simulink model "justina_control"  (R2020a)
settings: Solver=ode4  StartTime=0.0  StopTime=inf  FixedStep=0.004  MaxStep=0.01  RelTol=1e-3
PreLoadFcn:
  | load('justina_rigid_body_tree')
InitFcn:
  | [lowpass_B, lowpass_A] = butter(4,1,'s');
  | manipulator_tree = importrobot('justina_description.urdf');
  | manipulator_tree.Gravity = [9.81 0 0];
model workspace (MAT data in the model file):
  SL_ROS_VariableLengthArrays_MaxSizes.CommonInfo.ArrayTruncateAction = 'EmitWarning'
  SL_ROS_VariableLengthArrays_MaxSizes.MsgTypeMap = containers.Map
  SL_ROS_VariableLengthArrays_MaxSizes.MsgTypeMap.serialization.keys = {'sensor_msgs/JointState', 'std_msgs/Float32MultiArray', 'std_msgs/Float64MultiArray', 'std_msgs/String'}
  SL_ROS_VariableLengthArrays_MaxSizes.MsgTypeMap.serialization.values{1}(1).PropertyName = 'Effort'
  SL_ROS_VariableLengthArrays_MaxSizes.MsgTypeMap.serialization.values{1}(1).DataType = 'double'
  SL_ROS_VariableLengthArrays_MaxSizes.MsgTypeMap.serialization.values{1}(1).MaxLength = 7
  SL_ROS_VariableLengthArrays_MaxSizes.MsgTypeMap.serialization.values{1}(2).PropertyName = 'Name'
  SL_ROS_VariableLengthArrays_MaxSizes.MsgTypeMap.serialization.values{1}(2).DataType = 'std_msgs/String'
  SL_ROS_VariableLengthArrays_MaxSizes.MsgTypeMap.serialization.values{1}(2).MaxLength = 7
  SL_ROS_VariableLengthArrays_MaxSizes.MsgTypeMap.serialization.values{1}(3).PropertyName = 'Position'
  SL_ROS_VariableLengthArrays_MaxSizes.MsgTypeMap.serialization.values{1}(3).DataType = 'double'
  SL_ROS_VariableLengthArrays_MaxSizes.MsgTypeMap.serialization.values{1}(3).MaxLength = 7
  SL_ROS_VariableLengthArrays_MaxSizes.MsgTypeMap.serialization.values{1}(4).PropertyName = 'Velocity'
  SL_ROS_VariableLengthArrays_MaxSizes.MsgTypeMap.serialization.values{1}(4).DataType = 'double'
  SL_ROS_VariableLengthArrays_MaxSizes.MsgTypeMap.serialization.values{1}(4).MaxLength = 7
  SL_ROS_VariableLengthArrays_MaxSizes.MsgTypeMap.serialization.values{2}.PropertyName = 'Data'
  SL_ROS_VariableLengthArrays_MaxSizes.MsgTypeMap.serialization.values{2}.DataType = 'single'
  SL_ROS_VariableLengthArrays_MaxSizes.MsgTypeMap.serialization.values{2}.MaxLength = 14
  SL_ROS_VariableLengthArrays_MaxSizes.MsgTypeMap.serialization.values{3}.PropertyName = 'Data'
  SL_ROS_VariableLengthArrays_MaxSizes.MsgTypeMap.serialization.values{3}.DataType = 'double'
  SL_ROS_VariableLengthArrays_MaxSizes.MsgTypeMap.serialization.values{3}.MaxLength = 7
  SL_ROS_VariableLengthArrays_MaxSizes.MsgTypeMap.serialization.values{4}.PropertyName = 'Data'
  SL_ROS_VariableLengthArrays_MaxSizes.MsgTypeMap.serialization.values{4}.DataType = 'uint8'
  SL_ROS_VariableLengthArrays_MaxSizes.MsgTypeMap.serialization.values{4}.MaxLength = 10
  SL_ROS_VariableLengthArrays_MaxSizes.MsgTypeMap.serialization.uniformity = 0
  SL_ROS_VariableLengthArrays_MaxSizes.MsgTypeMap.serialization.keyType = 'char'
  SL_ROS_VariableLengthArrays_MaxSizes.MsgTypeMap.serialization.valueType = 'any'
undefined symbols (not defined in the file or in its folder): Data, Data_SL_Info
libraries: robotlib x19, robotmaniplib x1
settings Model: EnablePacing=on  Creator=marco  LastModifiedBy=josea
settings OptimizationCC: EnhancedBackFolding=on  PassReuseOutputArgsAs=Individual arguments  ZeroExternalMemoryAtStartup=off  ZeroInternalMemoryAtStartup=off  MaxStackSize=64  OptimizeBlockOrder=speed  DifferentSizesBufferReuse=on  OptimizationCustomize=off  EfficientTunableParamExpr=on
settings DebuggingCC: ParameterTunabilityLossMsg=error
settings HardwareCC: ProdBitPerLong=64  ProdHWDeviceType=Intel->x86-64 (Linux 64)
settings SFSimCC: CustomCodeUndefinedFunction=ThrowError
settings RTWCC: SystemTargetFile=ert.tlc  HardwareBoard=Robot Operating System (ROS)  TemplateMakefile=ert_default_tmf  GenerateReport=on  Toolchain=Catkin  IncludeHyperlinkInReport=on  LaunchReport=on  TargetLang=C++  GenerateTraceInfo=on  GenerateTraceReport=on  GenerateTraceReportSl=on  GenerateTraceReportSf=on  GenerateTraceReportEml=on
settings CodeAppCC: ForceParamTrailComments=on  IgnoreCustomStorageClasses=off  OperatorAnnotations=on  SimulinkDataObjDesc=on  SFDataObjDesc=on  InsertBlockDesc=on
settings ERTTargetCC: SupportContinuousTime=on  SupportVariableSizeSignals=on
settings ExplorerConfigSet: InternalSimMechanicsExplorerSettings="<ExplorerConfiguration><canonicalview>aerospace</canonicalview><AnimationSetting><BasePlaybackSpeed>1.0</BasePlaybackSpeed><PlaybackSpeedFactor>1.0</PlaybackSpeedFactor></AnimationSetting><TilePanel><TileInfo><Tiles Columns=\"1\" Count=\"1\" Rows=\"1\"><Column Weight=\"1\"/><Row Weight=\"1\"/><Tile Height=\"1\" Width=\"1\" X=\"0\" Y=\"0\"/></Tiles></TileInfo><SceneInfo><SceneViewer><BGColor><R>0.60000002384185791</R><G>0.60000002384185791</G><B>0.60000002384185791</B></BGColor><Camera><DoPerspective>off</DoPerspective><Position><X>0.470747241724220999</X><Y>0.672742710715300452</Y><Z>0.803552756362765797</Z></Position><Center><X>0.426167977285198674</X><Y>0.0857009724355916047</Y><Z>-0.00477557216445684274</Z></Center><Up><X>-0.998971998504803671</X><Y>0.0328560329609175472</Y><Z>0.0312318315407420499</Z></Up><ViewLimDist>1</ViewLimDist><YLim>0.446111832261085528</YLim><XLim>0.664557689711664734</XLim></Camera></SceneViewer></SceneInfo></TilePanel><MechEditorPanel><Cameras/><GfxPanelCameraMap/><VideoCreator><PlaybackSpeedRatio>1.0</PlaybackSpeedRatio><FrameRate>30</FrameRate><VideoFormat>Motion JPEG AVI</VideoFormat><FrameSize>auto</FrameSize></VideoCreator></MechEditorPanel></ExplorerConfiguration>"

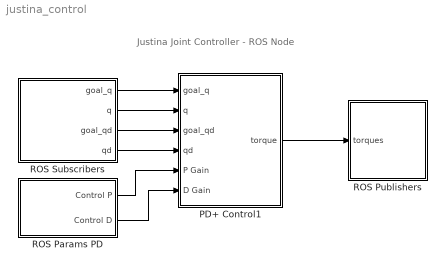
== system justina_control ==
  note: Justina Joint Controller - ROS Node
  PD+ Control1 : Subsystem
  ROS Params PD : Subsystem
  ROS Publishers : Subsystem
  ROS Subscribers : Subsystem
  wires:
  ROS Subscribers/1(goal_q) -> PD+ Control1/1(goal_q)
  ROS Subscribers/2(q) -> PD+ Control1/2(q)
  ROS Subscribers/3(goal_qd) -> PD+ Control1/3(goal_qd)
  ROS Subscribers/4(qd) -> PD+ Control1/4(qd)
  ROS Params PD/1(Control P) -> PD+ Control1/5(P Gain)
  ROS Params PD/2(Control D) -> PD+ Control1/6(D Gain)
  PD+ Control1/1(torque) -> ROS Publishers/1(torques)

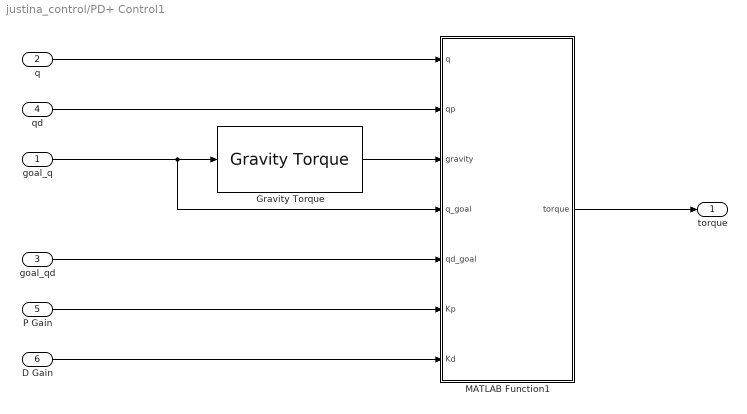
== system justina_control/PD+ Control1 ==
  goal_q : Inport
  q : Inport  Port=2
  goal_qd : Inport  Port=3
  qd : Inport  Port=4
  P Gain : Inport  Port=5
  D Gain : Inport  Port=6
  Gravity Torque : robotmaniplib/Gravity Torque  RigidBodyTree=manipulator_tree  SimulateUsing=Code generation
  MATLAB Function1 : MATLAB Function  TreatAsAtomicUnit=on
  torque : Outport
  wires:
  D Gain/1 -> MATLAB Function1/7(Kd)
  P Gain/1 -> MATLAB Function1/6(Kp)
  q/1 -> MATLAB Function1/1(q)
  qd/1 -> MATLAB Function1/2(qp)
  goal_qd/1 -> MATLAB Function1/5(qd_goal)
  goal_q/1 -> Gravity Torque/1, MATLAB Function1/4(q_goal)
  MATLAB Function1/1(torque) -> torque/1
  Gravity Torque/1 -> MATLAB Function1/3(gravity)

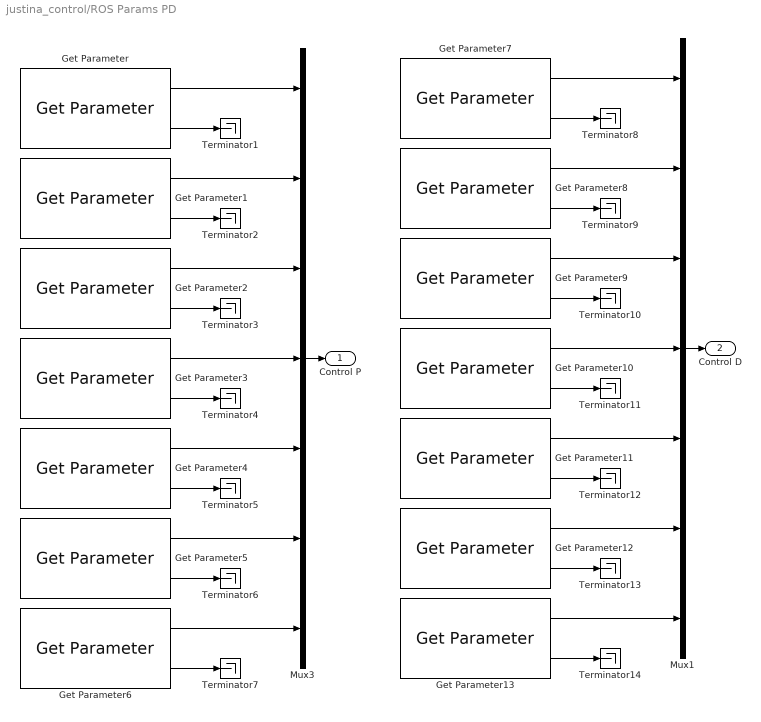
== system justina_control/ROS Params PD ==
  Get Parameter : robotlib/Get Parameter  ParameterSource=Specify your own  ParameterName=/control/P1  ParameterType=double  ParameterMaxArrayLength=16  ParameterInitialValue=0.0  SampleTime=1  ShowErrorCodeOutput=on  ModelName=justina_control  BlockId=ParamGet_justina_control_368
      settings: SourceProductBaseCode=RR
  Get Parameter1 : robotlib/Get Parameter  ParameterSource=Specify your own  ParameterName=/control/P2  ParameterType=double  ParameterMaxArrayLength=16  ParameterInitialValue=0.0  SampleTime=1  ShowErrorCodeOutput=on  ModelName=justina_control  BlockId=ParamGet_justina_control_370
      settings: SourceProductBaseCode=RR
  Get Parameter10 : robotlib/Get Parameter  ParameterSource=Specify your own  ParameterName=/control/D4  ParameterType=double  ParameterMaxArrayLength=16  ParameterInitialValue=0.0  SampleTime=1  ShowErrorCodeOutput=on  ModelName=justina_control  BlockId=ParamGet_justina_control_403
      settings: SourceProductBaseCode=RR
  Get Parameter11 : robotlib/Get Parameter  ParameterSource=Specify your own  ParameterName=/control/D5  ParameterType=double  ParameterMaxArrayLength=16  ParameterInitialValue=0.0  SampleTime=1  ShowErrorCodeOutput=on  ModelName=justina_control  BlockId=ParamGet_justina_control_404
      settings: SourceProductBaseCode=RR
  Get Parameter12 : robotlib/Get Parameter  ParameterSource=Specify your own  ParameterName=/control/D6  ParameterType=double  ParameterMaxArrayLength=16  ParameterInitialValue=0.0  SampleTime=1  ShowErrorCodeOutput=on  ModelName=justina_control  BlockId=ParamGet_justina_control_405
      settings: SourceProductBaseCode=RR
  Get Parameter13 : robotlib/Get Parameter  ParameterSource=Specify your own  ParameterName=/control/D7  ParameterType=double  ParameterMaxArrayLength=16  ParameterInitialValue=0.0  SampleTime=1  ShowErrorCodeOutput=on  ModelName=justina_control  BlockId=ParamGet_justina_control_406
      settings: SourceProductBaseCode=RR
  Get Parameter2 : robotlib/Get Parameter  ParameterSource=Specify your own  ParameterName=/control/P3  ParameterType=double  ParameterMaxArrayLength=16  ParameterInitialValue=0.0  SampleTime=1  ShowErrorCodeOutput=on  ModelName=justina_control  BlockId=ParamGet_justina_control_372
      settings: SourceProductBaseCode=RR
  Get Parameter3 : robotlib/Get Parameter  ParameterSource=Specify your own  ParameterName=/control/P4  ParameterType=double  ParameterMaxArrayLength=16  ParameterInitialValue=0.0  SampleTime=1  ShowErrorCodeOutput=on  ModelName=justina_control  BlockId=ParamGet_justina_control_374
      settings: SourceProductBaseCode=RR
  Get Parameter4 : robotlib/Get Parameter  ParameterSource=Specify your own  ParameterName=/control/P5  ParameterType=double  ParameterMaxArrayLength=16  ParameterInitialValue=0.0  SampleTime=1  ShowErrorCodeOutput=on  ModelName=justina_control  BlockId=ParamGet_justina_control_376
      settings: SourceProductBaseCode=RR
  Get Parameter5 : robotlib/Get Parameter  ParameterSource=Specify your own  ParameterName=/control/P6  ParameterType=double  ParameterMaxArrayLength=16  ParameterInitialValue=0.0  SampleTime=1  ShowErrorCodeOutput=on  ModelName=justina_control  BlockId=ParamGet_justina_control_378
      settings: SourceProductBaseCode=RR
  Get Parameter6 : robotlib/Get Parameter  ParameterSource=Specify your own  ParameterName=/control/P7  ParameterType=double  ParameterMaxArrayLength=16  ParameterInitialValue=0.0  SampleTime=1  ShowErrorCodeOutput=on  ModelName=justina_control  BlockId=ParamGet_justina_control_380
      settings: SourceProductBaseCode=RR
  Get Parameter7 : robotlib/Get Parameter  ParameterSource=Specify your own  ParameterName=/control/D1  ParameterType=double  ParameterMaxArrayLength=16  ParameterInitialValue=0.0  SampleTime=1  ShowErrorCodeOutput=on  ModelName=justina_control  BlockId=ParamGet_justina_control_400
      settings: SourceProductBaseCode=RR
  Get Parameter8 : robotlib/Get Parameter  ParameterSource=Specify your own  ParameterName=/control/D2  ParameterType=double  ParameterMaxArrayLength=16  ParameterInitialValue=0.0  SampleTime=1  ShowErrorCodeOutput=on  ModelName=justina_control  BlockId=ParamGet_justina_control_401
      settings: SourceProductBaseCode=RR
  Get Parameter9 : robotlib/Get Parameter  ParameterSource=Specify your own  ParameterName=/control/D3  ParameterType=double  ParameterMaxArrayLength=16  ParameterInitialValue=0.0  SampleTime=1  ShowErrorCodeOutput=on  ModelName=justina_control  BlockId=ParamGet_justina_control_402
      settings: SourceProductBaseCode=RR
  Mux1 : Mux  Inputs=7
  Mux3 : Mux  Inputs=7
  Terminator{1..14} (14 alike) : Terminator
  Control P : Outport
  Control D : Outport  Port=2
  wires:
  Get Parameter5/1 -> Mux3/6
  Get Parameter7/1 -> Mux1/1
  Get Parameter12/1 -> Mux1/6
  Get Parameter13/2 -> Terminator14/1
  Get Parameter13/1 -> Mux1/7
  Get Parameter2/1 -> Mux3/3
  Get Parameter11/2 -> Terminator12/1
  Get Parameter/1 -> Mux3/1
  Get Parameter12/2 -> Terminator13/1
  Get Parameter3/1 -> Mux3/4
  Get Parameter/2 -> Terminator1/1
  Get Parameter4/1 -> Mux3/5
  Get Parameter6/2 -> Terminator7/1
  Get Parameter10/1 -> Mux1/4
  Get Parameter6/1 -> Mux3/7
  Get Parameter9/2 -> Terminator10/1
  Get Parameter2/2 -> Terminator3/1
  Get Parameter7/2 -> Terminator8/1
  Mux1/1 -> Control D/1
  Get Parameter1/2 -> Terminator2/1
  Get Parameter5/2 -> Terminator6/1
  Get Parameter1/1 -> Mux3/2
  Get Parameter8/1 -> Mux1/2
  Get Parameter8/2 -> Terminator9/1
  Get Parameter10/2 -> Terminator11/1
  Get Parameter4/2 -> Terminator5/1
  Get Parameter3/2 -> Terminator4/1
  Mux3/1 -> Control P/1
  Get Parameter9/1 -> Mux1/3
  Get Parameter11/1 -> Mux1/5

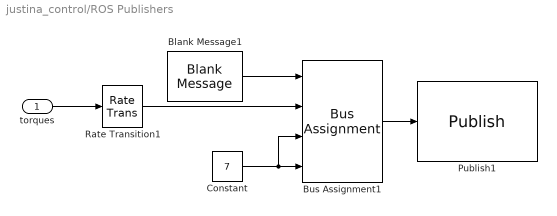
== system justina_control/ROS Publishers ==
  torques : Inport
  Blank Message1 : robotlib/Blank Message  messageClass=Message  entityType=std_msgs/Float64MultiArray  messageType=std_msgs/Float64MultiArray  SampleTime=0.004
  Bus Assignment1 : BusAssignment  AssignedSignals=Data,Data_SL_Info.CurrentLength,Data_SL_Info.ReceivedLength
  Constant : Constant  Value=7  OutDataTypeStr=uint32  SampleTime=0.004
  Publish1 : robotlib/Publish  topicSource=Specify your own  topic=/joint_torques  messageType=std_msgs/Float64MultiArray  messageQueueLength=1
  Rate Transition1 : RateTransition
  wires:
  Blank Message1/1 -> Bus Assignment1/1
  Rate Transition1/1 -> Bus Assignment1/2
  torques/1 -> Rate Transition1/1
  Bus Assignment1/1 -> Publish1/1
  Constant/1 -> Bus Assignment1/4, Bus Assignment1/3

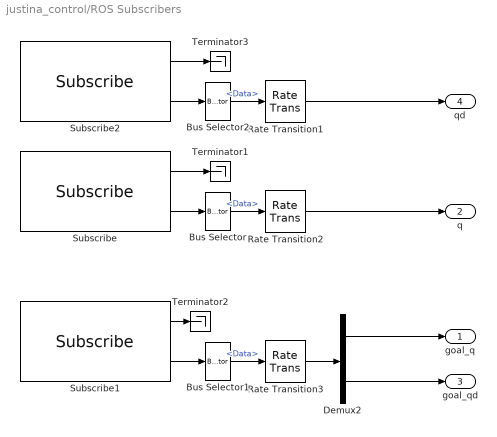
== system justina_control/ROS Subscribers ==
  Bus Selector : BusSelector  OutputSignals=Data
  Bus Selector1 : BusSelector  OutputSignals=Data
  Bus Selector2 : BusSelector  OutputSignals=Data
  Demux2 : Demux  Outputs=[7,7]
  Rate Transition1 : RateTransition
  Rate Transition2 : RateTransition
  Rate Transition3 : RateTransition
  Subscribe : robotlib/Subscribe  topicSource=Specify your own  topic=/joint_positions  messageType=std_msgs/Float64MultiArray  sampleTime=0.004  messageQueueLength=1
  Subscribe1 : robotlib/Subscribe  topicSource=Specify your own  topic=/goal_trajectory  messageType=std_msgs/Float32MultiArray  sampleTime=0.004  messageQueueLength=1
  Subscribe2 : robotlib/Subscribe  topicSource=Specify your own  topic=/joint_speeds  messageType=std_msgs/Float64MultiArray  sampleTime=0.004  messageQueueLength=1
  Terminator1 : Terminator
  Terminator2 : Terminator
  Terminator3 : Terminator
  goal_q : Outport
  q : Outport  Port=2
  goal_qd : Outport  Port=3
  qd : Outport  Port=4
  wires:
  Subscribe1/1 -> Terminator2/1
  Subscribe1/2 -> Bus Selector1/1
  Bus Selector/1 -> Rate Transition2/1  "<Data>"
  Rate Transition2/1 -> q/1
  Demux2/1 -> goal_q/1
  Subscribe/2 -> Bus Selector/1
  Rate Transition3/1 -> Demux2/1
  Demux2/2 -> goal_qd/1
  Bus Selector1/1 -> Rate Transition3/1  "<Data>"
  Subscribe/1 -> Terminator1/1
  Subscribe2/2 -> Bus Selector2/1
  Subscribe2/1 -> Terminator3/1
  Bus Selector2/1 -> Rate Transition1/1  "<Data>"
  Rate Transition1/1 -> qd/1

== matlab function justina_control/PD+ Control1/MATLAB Function1 ==
  data: q input; qp input; gravity input; q_goal input; torque output; qd_goal input; Kp input; Kd input
function torque = position_control(q,qp, gravity, q_goal, qd_goal, Kp, Kd)
%%Constantes del control PD

qe = zeros(1,7);
qpe = zeros(1,7);
torque = zeros(1,7);
for i=1:7
    qe(i) = q_goal(i) - q(i);
    qpe(i) = qd_goal(i) - qp(i);
    torque(i) = gravity(i) + Kp(i)*qe(i) + Kd(i)*qpe(i);
    if torque(i) > 2.5
        torque(i) = 2.5;
    elseif torque(i) < -2.5
        torque(i) = -2.5;
    end
end
